simulink model "statemachine1"  (R2025a)
settings: Solver=VariableStepAuto  StartTime=0.0  StopTime=10.0  RelTol=1e-3
settings Model: Creator=harri  LastModifiedBy=harri

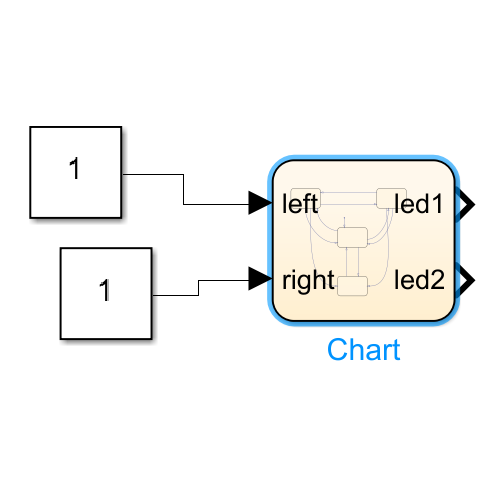
[thumbnail: Simulink's stored preview of the top-level diagram]
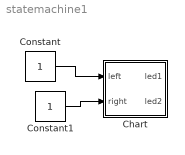
== system statemachine1 ==
  Chart : Stateflow chart  TreatAsAtomicUnit=on
  Constant : Constant
  Constant1 : Constant
  wires:
  Constant/1 -> Chart/1(left)
  Constant1/1 -> Chart/2(right)

== stateflow chart statemachine1/Chart ==
  state LED_ON
    entry:
    led1 = 1;
    led2 = 0;
  state RIGHT_ON
    entry:
    led1 = 0;
    led2 = 1;
  state OFF
    entry:
    led1 = 0;
    led2 = 0;
  state HAZARD
    entry:
    led1 = 1;
    led2 = 1;
  RIGHT_ON -> LED_ON [order 1] : [left == 1 && right == 0]
  LED_ON -> RIGHT_ON [order 1] : [left == 0 && right == 1]
  LED_ON -> OFF [order 2] : [left == 1 && right == 0]
  LED_ON -> HAZARD [order 3] : [left == 1 && right == 1]
  OFF -> LED_ON [order 3] : [left == 1 && right == 0]
  OFF -> RIGHT_ON [order 2] : [left == 0 && right == 1]
  RIGHT_ON -> OFF [order 2] : [left == 0 && right == 1]
  RIGHT_ON -> HAZARD [order 3] : [left == 1 && right == 1]
  (default) -> OFF
  HAZARD -> OFF : [left == 0 || right == 0]
  OFF -> HAZARD [order 1] : [left == 1 && right == 1]
  data: left input; right input; led1 output; led2 output
